simulink model "Torque_Transformation"  (R2016a)
settings: Solver=FixedStepAuto  SolverMode=SingleTasking  StartTime=0.0  StopTime=10  RelTol=1e-3
values from neighbouring files (symbols this model uses):
  alpha = pi/4    (= 0.785398163397)    [Parameters_ETHZ.m]    (also in Parameters_Geschaetzt.m; Parameters_Group.m; Parameters_Twente.m)
  beta = 0    [Parameters_ETHZ.m]    (also in Parameters_Geschaetzt.m = 4.18879020479; Parameters_Group.m = 1.0471975512; Parameters_Twente.m)
settings Model: Creator=Florian  LastModifiedBy=Florian
settings OptimizationCC: DefaultParameterBehavior=Inlined  UseDivisionForNetSlopeComputation=on  UseFloatMulNetSlope=on  InlineInvariantSignals=on  PassReuseOutputArgsAs=Individual arguments  ZeroExternalMemoryAtStartup=off  ZeroInternalMemoryAtStartup=off  NoFixptDivByZeroProtection=on  EfficientFloat2IntCast=on  OptimizeModelRefInitCode=on  LifeSpan=1
settings HardwareCC: ProdBitPerPointer=32  ProdLargestAtomicInteger=Long  ProdLargestAtomicFloat=Double  ProdWordSize=32  ProdHWDeviceType=ARM Compatible->ARM Cortex
settings RTWCC: SystemTargetFile=ert.tlc  TemplateMakefile=ert_default_tmf  GenerateReport=on  IncludeHyperlinkInReport=on  LaunchReport=on  GenerateTraceInfo=on  GenerateTraceReport=on  GenerateTraceReportSl=on  GenerateTraceReportSf=on  GenerateTraceReportEml=on  GenerateCodeMetricsReport=on
settings CodeAppCC: ForceParamTrailComments=on  IgnoreCustomStorageClasses=off  OperatorAnnotations=on  SimulinkDataObjDesc=on  SFDataObjDesc=on  MATLABFcnDesc=on  InsertBlockDesc=on  MATLABSourceComments=on
settings ERTTargetCC: GenerateSampleERTMain=on  IncludeMdlTerminateFcn=off  CombineSignalStateStructs=on  SupportComplex=off  SupportContinuousTime=on  InlinedParameterPlacement=NonHierarchical  ERTCustomFileTemplate=example_file_process.tlc  ERTFilePackagingFormat=CompactWithDataFile

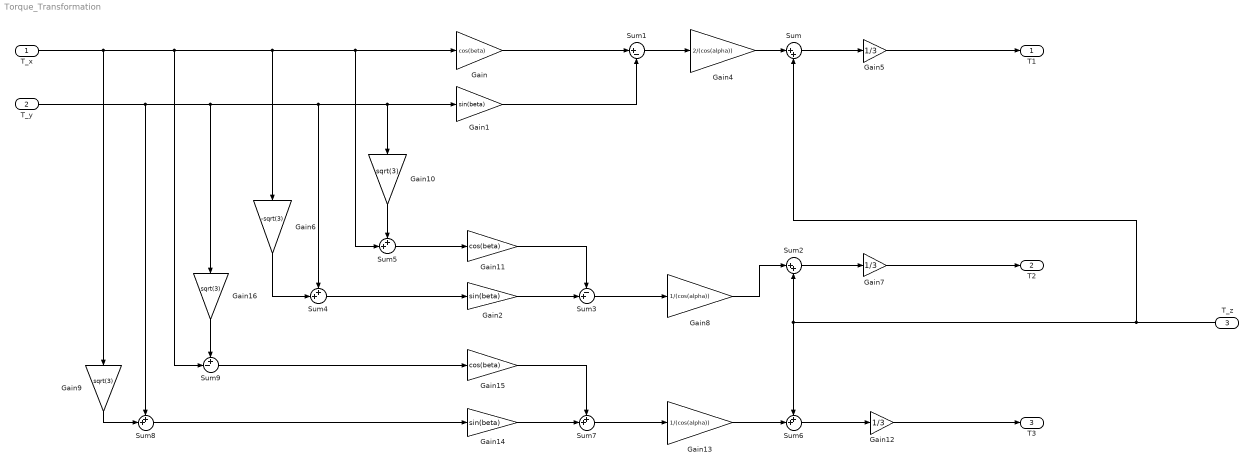
== system Torque_Transformation ==
  T_x : Inport
  T_y : Inport  Port=2
  T_z : Inport  Port=3
  Gain : Gain  Gain=cos(beta)
  Gain1 : Gain  Gain=sin(beta)
  Gain10 : Gain  Gain=sqrt(3)
  Gain11 : Gain  Gain=cos(beta)
  Gain12 : Gain  Gain=1/3
  Gain13 : Gain  Gain=1/(cos(alpha))
  Gain14 : Gain  Gain=sin(beta)
  Gain15 : Gain  Gain=cos(beta)
  Gain16 : Gain  Gain=sqrt(3)
  Gain2 : Gain  Gain=sin(beta)
  Gain4 : Gain  Gain=2/(cos(alpha))
  Gain5 : Gain  Gain=1/3
  Gain6 : Gain  Gain=-sqrt(3)
  Gain7 : Gain  Gain=1/3
  Gain8 : Gain  Gain=1/(cos(alpha))
  Gain9 : Gain  Gain=sqrt(3)
  Sum : Sum  Inputs=|++
  Sum1 : Sum  Inputs=|+-
  Sum2 : Sum  Inputs=|++
  Sum3 : Sum  Inputs=-+|
  Sum{4..8} (5 alike) : Sum  Inputs=++|
  Sum9 : Sum  Inputs=+-|
  T1 : Outport
  T2 : Outport  Port=2
  T3 : Outport  Port=3
  wires:
  Gain5/1 -> T1/1
  Sum/1 -> Gain5/1
  Gain4/1 -> Sum/1
  Sum1/1 -> Gain4/1
  T_x/1 -> Sum9/2, Gain/1, Sum5/2, Gain6/1, Gain9/1
  Gain/1 -> Sum1/1
  T_y/1 -> Gain16/1, Gain1/1, Gain10/1, Sum4/1, Sum8/1
  Gain1/1 -> Sum1/2
  Gain7/1 -> T2/1
  Sum2/1 -> Gain7/1
  Gain8/1 -> Sum2/1
  Sum3/1 -> Gain8/1
  Gain2/1 -> Sum3/2
  Sum4/1 -> Gain2/1
  Gain6/1 -> Sum4/2
  Gain11/1 -> Sum3/1
  Sum5/1 -> Gain11/1
  Gain10/1 -> Sum5/1
  Gain12/1 -> T3/1
  Sum6/1 -> Gain12/1
  Gain13/1 -> Sum6/2
  T_z/1 -> Sum2/2, Sum6/1, Sum/2
  Sum7/1 -> Gain13/1
  Sum8/1 -> Gain14/1
  Gain9/1 -> Sum8/2
  Gain14/1 -> Sum7/2
  Gain15/1 -> Sum7/1
  Gain16/1 -> Sum9/1
  Sum9/1 -> Gain15/1
